simulink model "Week1"  (R2023b)
settings: Solver=ode1  StartTime=0.0  StopTime=25  FixedStep=dT_current  RelTol=1e-3
values from neighbouring files (symbols this model uses):
  A = 1    [Week1_code.m]
  b = 1    [Week1_code.m]
  J = 1    [Week1_code.m]
  w_0 = 1.0    (= 1)    [Week1_code.m]
settings Model: Creator=jessi  LastModifiedBy=jessi

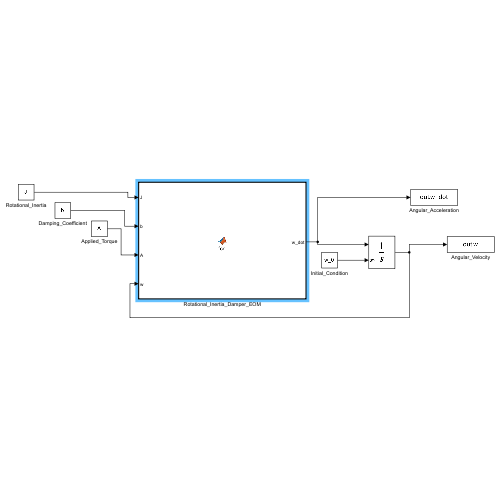
[thumbnail: Simulink's stored preview of the top-level diagram]
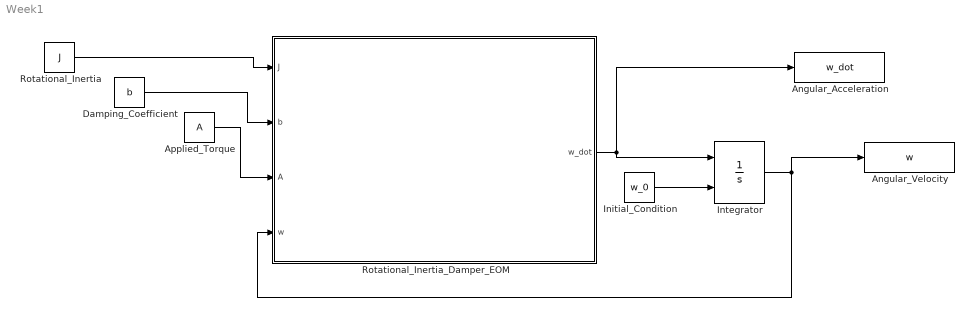
== system Week1 ==
  Angular_Acceleration : ToWorkspace  VariableName=w_dot  SaveFormat=Timeseries  SampleTime=-1
  Angular_Velocity : ToWorkspace  VariableName=w  SaveFormat=Timeseries  SampleTime=-1
  Applied_Torque : Constant  Value=A
  Damping_Coefficient : Constant  Value=b
  Initial_Condition : Constant  Value=w_0
  Integrator : Integrator  InitialConditionSource=external
  Rotational_Inertia : Constant  Value=J
  Rotational_Inertia_Damper_EOM : MATLAB Function  TreatAsAtomicUnit=on
  wires:
  Rotational_Inertia/1 -> Rotational_Inertia_Damper_EOM/1(J)
  Damping_Coefficient/1 -> Rotational_Inertia_Damper_EOM/2(b)
  Applied_Torque/1 -> Rotational_Inertia_Damper_EOM/3(A)
  Rotational_Inertia_Damper_EOM/1(w_dot) -> Angular_Acceleration/1, Integrator/1
  Initial_Condition/1 -> Integrator/2
  Integrator/1 -> Angular_Velocity/1, Rotational_Inertia_Damper_EOM/4(w)

== matlab function Week1/Rotational_Inertia_Damper_EOM ==
  data: J input; w_dot output; b input; A input; w input
function w_dot = fcn(J,b,A,w)


w_dot = (1/J)*(A-b*w);

end
